simulink model "PRE5"  (R2021a)
settings: Solver=ode23t  StartTime=0.0  StopTime=0.1  MaxStep=1e-6  RelTol=1e-3
libraries: dsparch4 x2, commsynccomp2 x1, spspowerguiLib x1
settings Model: Creator=Dell  LastModifiedBy=Dell

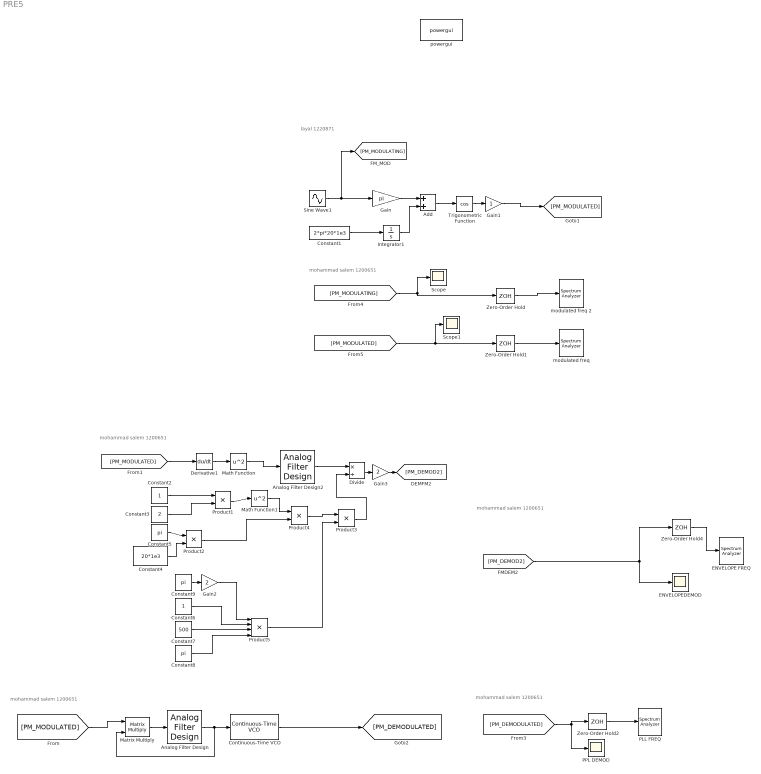
== system PRE5 ==
  note: layal 1220871
  note: mohammad salem 1200651
  note: mohammad salem 1200651
  note: mohammad salem 1200651
  note: mohammad salem 1200651
  note: mohammad salem 1200651
  Add : Sum
  Analog Filter Design : dsparch4/Analog Filter Design  method=Butterworth  filttype=Lowpass  N=4  Wlo=2*pi*20000  Whi=80  Rp=2  Rs=40
  Analog Filter Design2 : dsparch4/Analog Filter Design  method=Butterworth  filttype=Bandpass  N=4  Wlo=500  Whi=40500  Rp=2  Rs=40
  Constant1 : Constant  Value=2*pi*20*1e3
  Constant2 : Constant
  Constant3 : Constant  Value=2
  Constant4 : Constant  Value=20*1e3
  Constant5 : Constant  Value=pi
  Constant6 : Constant
  Constant7 : Constant  Value=500
  Constant8 : Constant  Value=pi
  Constant9 : Constant  Value=pi
  Continuous-Time VCO : commsynccomp2/Continuous-Time VCO  Ac=1  Fc=20000  Kc=20000  Ph=0
      settings: SourceProductBaseCode=CM
  Derivative1 : Derivative
  Divide : Product  Inputs=*/
  "ENVELOPE FREQ  " : SpectrumAnalyzer
  "ENVELOPEDEMOD " : Scope
  Gain : Gain  Gain=pi
  Gain1 : Gain
  Gain2 : Gain  Gain=2
  Gain3 : Gain  Gain=2
  Integrator1 : Integrator
  Math Function : Math  Operator=square  SaturateOnIntegerOverflow=on
  Math Function1 : Math  Operator=square  SaturateOnIntegerOverflow=on
  Matrix Multiply : Product  Multiplication=Matrix(*)
  "PLL FREQ " : SpectrumAnalyzer
  "PPL DEMOD " : Scope
  Product{1..4} (4 alike) : Product
  Product5 : Product  Inputs=4
  Scope : Scope
  Scope1 : Scope
  Sine Wave1 : Sin  Frequency=2*pi*500  Phase=pi/2  Samples=5  SampleTime=0
  Trigonometric Function : Trigonometry  Operator=cos
  Zero-Order Hold{,1..2,4} (4 alike) : ZeroOrderHold  SampleTime=-1
  "modulated freq " : SpectrumAnalyzer
  modulated freq 2 : SpectrumAnalyzer
  powergui : spspowerguiLib/powergui  Priority=1  SimulationMode=Continuous  SampleTime=50e-6  frequency=60  Iterations=50  frequencyindice=60  Pbase=100e6  ErrMax=1e-4  UnitsV=kV  UnitsW=MW  buscounter=0  FunctionMessages=off  echomessages=off  EnableUseOfTLC=off  CurrentSourceSwitches=off  DisableSnubberDevices=off  DisableRonSwitches=off  DisableVfSwitches=off  DisplayEquations=off  AutomaticDiscreteSolvers=off  SolverType=Tustin/Backward Euler (TBE)  Interpol=off  ExternalGateDelay=off  methode=off  Ts=100  x0status=blocks  SPID=on  SwTol=0  HookPort=off  NonlinearTolerance=1e-4  nMaxIteration=100  ContinueOnMaxIteration=off  RestoreLinks=warning  ResistiveCurrentMeasurement=off  Frange=[0:2:500]  Ylog=off  Xlog=on  ShowGrid=off  save=off  variable=ZData  structure=0  ZoomFFT=off  StartTime=0.0  cycles=1  DisplayStyle=1  fundamental=60  FreqAxis=off  MaxFrequency=1000  frequencyindicesteady=1  RmsSteady=1  display=off
  wires:
  Add/1 -> Trigonometric Function/1
  Sine Wave1/1 -> Gain/1, [PM_MODULATING]
  Gain/1 -> Add/1
  Trigonometric Function/1 -> Gain1/1
  Constant1/1 -> Integrator1/1
  Zero-Order Hold1/1 -> "modulated freq "/1
  Zero-Order Hold/1 -> modulated freq 2/1
  [PM_MODULATING] -> Zero-Order Hold/1, Scope/1
  Integrator1/1 -> Add/2
  [PM_DEMOD2] -> Zero-Order Hold4/1, "ENVELOPEDEMOD "/1
  Constant3/1 -> Product1/2
  Constant8/1 -> Product5/4
  Product3/1 -> Divide/2
  Math Function1/1 -> Product4/1
  Product1/1 -> Math Function1/1
  Constant2/1 -> Product1/1
  Math Function/1 -> Analog Filter Design2/1
  Constant7/1 -> Product5/3
  Derivative1/1 -> Math Function/1
  Zero-Order Hold4/1 -> "ENVELOPE FREQ  "/1
  [PM_MODULATED] -> Derivative1/1
  Analog Filter Design2/1 -> Divide/1
  Continuous-Time VCO/1 -> [PM_DEMODULATED]
  Analog Filter Design/1 -> Matrix Multiply/2, Continuous-Time VCO/1
  [PM_MODULATED] -> Matrix Multiply/1
  Zero-Order Hold2/1 -> "PLL FREQ "/1
  [PM_DEMODULATED] -> Zero-Order Hold2/1, "PPL DEMOD "/1
  Matrix Multiply/1 -> Analog Filter Design/1
  Constant5/1 -> Product2/1
  Constant4/1 -> Product2/2
  Product2/1 -> Product4/2
  Constant9/1 -> Gain2/1
  Gain2/1 -> Product5/1
  Constant6/1 -> Product5/2
  Product5/1 -> Product3/2
  Product4/1 -> Product3/1
  Divide/1 -> Gain3/1
  Gain3/1 -> [PM_DEMOD2]
  [PM_MODULATED] -> Zero-Order Hold1/1, Scope1/1
  Gain1/1 -> [PM_MODULATED]
